simulink model "VDCHyd2020a"  (R2020a)
settings: Solver=daessc  StartTime=0.0  StopTime=simulationEndTime  FixedStep=0.001  RelTol=1e-2
values from neighbouring files (symbols this model uses):
  Bc1_V = [0;0;0;0;0;0]    [initializeSimulationGP.m]
  filtDV = init2ndOrderLowPassFilter(35*2*pi,1,controller.dT)    [initializeLowPassFilters.m]
  filtEnc = init2ndOrderLowPassFilter(35*2*pi,1,controller.dT)    [initializeLowPassFilters.m]
undefined symbols (not defined in the file or in its folder): aux, B11_r_B11Tc1, B11_V, B11_Vr, B11Ftot_r, B12_r_B12Tc2, B12_Rot_Tc2, B12_U_Tc2, B12_V, B12_Vr, B12Ftot_r, B31_r_B31B41, B31_V, B31_Vr, B31FTot_r, B32_r_B32B42, B32_Rot_B42, B32_U_B42, B32_V, B32_Vr, B32FTot_r, B41_r_B41Tc1, B41_V, B41_Vr, B41FTot_r, B42_r_B42Tc2, B42_Rot_Tc2, B42_U_Tc2, B42_V, B42_Vr, B42FTot_r, B52_r_B52P32, B52_Rot_P32, B52_U_P32, B52_V, B52_Vr, B52Ftot_r, Bc1_r_Bc1B11, Bc1_r_Bc1B31, Bc1_Vr, Bc1FTot_r, Bc2_r_Bc2B12, Bc2_r_Bc2B32, Bc2_Rot_B12, Bc2_Rot_B32, Bc2_U_B12, Bc2_U_B32, Bc2_V, Bc2_Vr, Bc2Tot_r, controller, cyl1, cyl2, cylT2, D22_V, D22_Vr, D22Fr, DiscIntNeverNeededParam, dq1, dq11 ... (+125)
libraries: sm_lib x34, nesl_utility x15, simulink x11, dspinverses x1
(part 12 of 12)

== matlab function VDCHyd2020a/sbVDCController/sbFormingControlActions/controlVoltageRS1 ==
  data: uf1r input; pS input; pR input; pa1 input; pb1 input; x1 input; thetav1 input; u1 output; hosing1 parameter; cyl1 parameter
function u1  = calculateControlVoltage(uf1r, pS, pR, pa1, pb1, x1, thetav1, hosing1, cyl1)

    cp1 = thetav1(1); cn1=thetav1(2); cp2=thetav1(3); cn2=thetav1(4);

    % Implemented per (27) in S. Lampinen, J. Koivumäki and J. Mattila, 
    % "Improved Hydraulic Cylinder Model for the Virtual Decomposition 
    % Control Approach," 2019 IEEE International Conference on Cybernetics 
    % and Intelligent Systems (CIS) and IEEE Conference on Robotics, 
    % Automation and Mechatronics (RAM), Bangkok, Thailand, 2019, 
    % pp. 113-118, doi: 10.1109/CIS-RAM47153.2019.9095788 
    u1 = uf1r*selFcn(uf1r)/( (cp1*sqAbsPresDrop(pS-pa1))/(hosing1.V0a/cyl1.Aa + x1) + (cn2*sqAbsPresDrop(pb1-pR))/(hosing1.V0b/cyl1.Ab + cyl1.sp - x1) ) + ...
         uf1r*selFcn(-uf1r)/( (cp2*sqAbsPresDrop(pS-pb1))/(hosing1.V0b/cyl1.Ab + cyl1.sp - x1) + (cn1*sqAbsPresDrop(pa1-pR))/(hosing1.V0a/cyl1.Aa + x1) );


end


function S = selFcn(U)

    if U > 0
        S = 1;
    else
        S = 0;
    end
    
end

function nup = sqAbsPresDrop(dp)

    nup = sign(dp)*sqrt(abs(dp));

end

== matlab function VDCHyd2020a/sbVDCController/sbFormingControlActions/regressorYd1 ==
  data: dfp1r input; Yd1 output; x1 input; dx1 input; pa1 input; pb1 input; hosing1 parameter; cyl1 parameter
function Yd1 = cylinderRegressor(dfp1r, x1, dx1, pa1, pb1, hosing1, cyl1)

    % Implemented per (43) in S. Lampinen, J. Koivumäki and J. Mattila, 
    % "Improved Hydraulic Cylinder Model for the Virtual Decomposition 
    % Control Approach," 2019 IEEE International Conference on Cybernetics 
    % and Intelligent Systems (CIS) and IEEE Conference on Robotics, 
    % Automation and Mechatronics (RAM), Bangkok, Thailand, 2019, 
    % pp. 113-118, doi: 10.1109/CIS-RAM47153.2019.9095788.
    Yd1 = [dfp1r,...
           dx1/(hosing1.V0a/cyl1.Aa + x1),...
           dx1/(hosing1.V0b/cyl1.Ab + cyl1.sp - x1),...
           ((pa1-pb1)*(cyl1.Aa*hosing1.V0b + cyl1.Ab*hosing1.V0a + cyl1.Aa*cyl1.Ab*cyl1.sp))/((hosing1.V0a + cyl1.Aa*x1)*(hosing1.V0b + cyl1.Ab*(cyl1.sp - x1)))];

end

== matlab function VDCHyd2020a/sbVDCController/sbFormingControlActions/regressorYvt2 ==
  data: ut2 input; Yvt2 output; pS input; pR input; pat2 input; pbt2 input; xt2 input; hosingT2 parameter; cylT2 parameter
function Yvt2 = valveRegressor(ut2, pS, pR, pat2, pbt2, xt2, hosingT2, cylT2)

    % Implemented per (25) in S. Lampinen, J. Koivumäki and J. Mattila, 
    % "Improved Hydraulic Cylinder Model for the Virtual Decomposition 
    % Control Approach," 2019 IEEE International Conference on Cybernetics 
    % and Intelligent Systems (CIS) and IEEE Conference on Robotics, 
    % Automation and Mechatronics (RAM), Bangkok, Thailand, 2019, 
    % pp. 113-118, doi: 10.1109/CIS-RAM47153.2019.9095788 in order
    % Yv = [cp1, cn1, cp2, cn2]
    Yvt2 = [sqAbsPresDrop(pS - pat2)*selFcn(ut2)*ut2/(hosingT2.V0a/cylT2.Aa + xt2),...
            sqAbsPresDrop(pat2 - pR)*selFcn(-ut2)*ut2/(hosingT2.V0a/cylT2.Aa + xt2),...
            sqAbsPresDrop(pS - pbt2)*selFcn(-ut2)*ut2/(hosingT2.V0b/cylT2.Ab + cylT2.sp - xt2),...
            sqAbsPresDrop(pbt2 - pR)*selFcn(ut2)*ut2/(hosingT2.V0b/cylT2.Ab + cylT2.sp - xt2)];

end

function S = selFcn(U)

    if U > 0
        S = 1;
    else
        S = 0;
    end
    
end

function nup = sqAbsPresDrop(dp)

    nup = sign(dp)*sqrt(abs(dp));

end

== matlab function VDCHyd2020a/sbVDCController/sbFormingControlActions/regressorYd2 ==
  data: dfp2r input; Yd2 output; x2 input; dx2 input; pa2 input; pb2 input; hosing2 parameter; cyl2 parameter
function Yd2 = cylinderRegressor(dfp2r, x2, dx2, pa2, pb2, hosing2, cyl2)
    
    % Implemented per (43) in S. Lampinen, J. Koivumäki and J. Mattila, 
    % "Improved Hydraulic Cylinder Model for the Virtual Decomposition 
    % Control Approach," 2019 IEEE International Conference on Cybernetics 
    % and Intelligent Systems (CIS) and IEEE Conference on Robotics, 
    % Automation and Mechatronics (RAM), Bangkok, Thailand, 2019, 
    % pp. 113-118, doi: 10.1109/CIS-RAM47153.2019.9095788.
    Yd2 = [dfp2r,...
           dx2/(hosing2.V0a/cyl2.Aa + x2),...
           dx2/(hosing2.V0b/cyl2.Ab + cyl2.sp - x2),...
           ((pa2-pb2)*(cyl2.Aa*hosing2.V0b + cyl2.Ab*hosing2.V0a + cyl2.Aa*cyl2.Ab*cyl2.sp))/((hosing2.V0a + cyl2.Aa*x2)*(hosing2.V0b + cyl2.Ab*(cyl2.sp - x2)))];

end
